simulink model "DynamicModel"  (R2023b)
settings: Solver=VariableStepAuto  StartTime=0.0  StopTime=25  RelTol=1e-3
InitFcn:
  | rho_inf = 1.22; % [kg/m^3] Air Density at sea level
  | C_d = 0.7; % [Non-Dimensional] **Guessed** Coefficient of Drag
  | R_air = 287; % [J/kg*K] Universal Gas Constant **Not used currently"
  | m = 6.8; % [kg] Total System Mass
  | g = 9.807; % [kg]
  | W = m * g; % [N] System Weight - Force of Gravity on system
  | D_p = 1.83; % [m] Diameter of Parachute Profile
  | S_p = (pi/4)*(D_p^2); % [m^2] Surface area of parachute profile
  | l_cp = 2; % [m] Distance from x_cp to the center of mass
  | 
  | % Motion Equation
  | a_33 = (4/3)*pi*(D_p/2)^3; % Motion along Z-Axis
  | a_11 = (1/2)*a_33; % Motion along X-Axis
  | a_22 = (1/2)*a_33; % Motion along Y-Axis
  | 
  | a_44 = l_cp*D_p^2*a_11; % Motion about the X-Axis
  | a_55 = l_cp*D_p^2*a_11; % Motion about the Y-Axis
  | 
  | fpa = rad2deg(90);
  | hdg = rad2deg(0);
settings Model: Creator=Blind  LastModifiedBy=Blind
settings DataIOCC: Refine=10

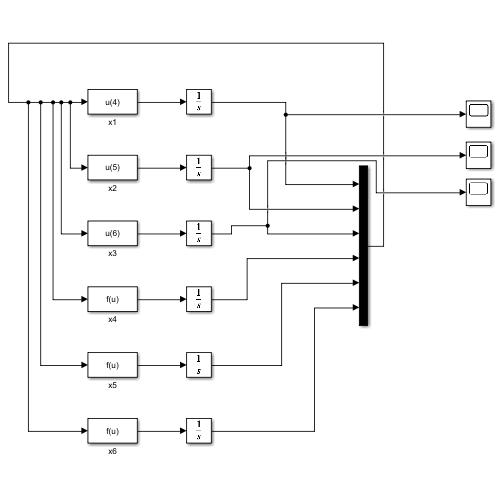
[thumbnail: Simulink's stored preview of the top-level diagram]
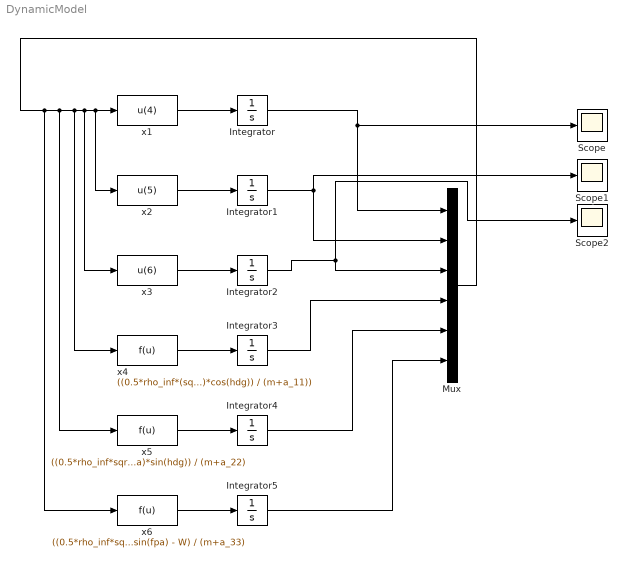
== system DynamicModel ==
  Integrator{,1..5} (6 alike) : Integrator
  Mux : Mux  Inputs=6
  Scope : Scope
  Scope1 : Scope
  Scope2 : Scope
  x1 : Fcn  Expr=u(4)
  x2 : Fcn  Expr=u(5)
  x3 : Fcn  Expr=u(6)
  x4 : Fcn  Expr=((0.5*rho_inf*(sqrt(u(4)^2+u(5)^2+u(6)^2))^2*cos(fpa)*cos(hdg)) / (m+a_11))
  x5 : Fcn  Expr=((0.5*rho_inf*sqrt(u(4)^2+u(5)^2+u(6)^2))^2*cos(fpa)*sin(hdg)) / (m+a_22)
  x6 : Fcn  Expr=((0.5*rho_inf*sqrt(u(4)^2+u(5)^2+u(6)^2))^2*sin(fpa) - W) / (m+a_33)
  wires:
  x1/1 -> Integrator/1
  x2/1 -> Integrator1/1
  x3/1 -> Integrator2/1
  x4/1 -> Integrator3/1
  x5/1 -> Integrator4/1
  x6/1 -> Integrator5/1
  Integrator/1 -> Scope/1, Mux/1
  Integrator1/1 -> Mux/2, Scope1/1
  Integrator2/1 -> Scope2/1, Mux/3
  Integrator4/1 -> Mux/5
  Integrator5/1 -> Mux/6
  Mux/1 -> x6/1, x5/1, x4/1, x3/1, x2/1, x1/1
  Integrator3/1 -> Mux/4
